simulink model "TEST1"  (R2023b)
settings: Solver=VariableStepAuto  StartTime=0.0  StopTime=10.0  RelTol=1e-3
libraries: spsExcitationSystemLib x2, spsMultiBandPowerSystemStabilizerLib x2, spsSynchronousMachinepuStandardLib x2, spsSteamTurbineandGovernorLib x2, spsThreePhaseTransformerTwoWindingsLib x2, spsThreePhasePISectionLineLib x2, spsThreePhaseParallelRLCLoadLib x1, sps_lib x1
settings Model: Creator=rohith  LastModifiedBy=rohith

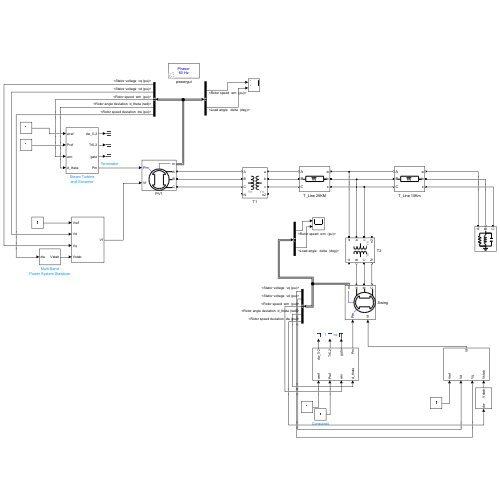
[thumbnail: Simulink's stored preview of the top-level diagram]
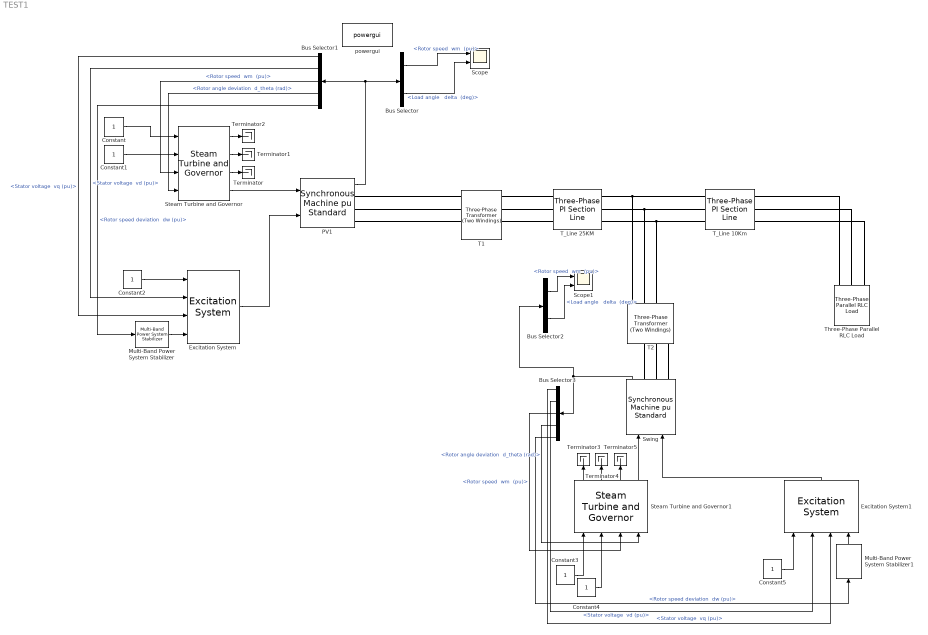
== system TEST1 ==
  Bus Selector : BusSelector  OutputSignals="Mechanical.Rotor speed  wm  (pu),Load angle   delta  (deg)"
  Bus Selector1 : BusSelector  OutputSignals="dq0 components.Stator voltage  vq (pu),dq0 components.Stator voltage  vd (pu),Mechanical.Rotor speed  wm  (pu),Mechanical.Rotor angle deviation  d_theta (rad),Mechanical.Rotor speed deviation  dw (pu)"
  Bus Selector2 : BusSelector  OutputSignals="Mechanical.Rotor speed  wm  (pu),Load angle   delta  (deg)"
  Bus Selector3 : BusSelector  OutputSignals="dq0 components.Stator voltage  vq (pu),dq0 components.Stator voltage  vd (pu),Mechanical.Rotor speed  wm  (pu),Mechanical.Rotor angle deviation  d_theta (rad),Mechanical.Rotor speed deviation  dw (pu)"
  Constant{,1..5} (6 alike) : Constant
  Excitation System : spsExcitationSystemLib/Excitation System  tr=20e-3  reg=[ 300, 0.001 ]  exc=[ 1, 0 ]  tgr=[ 0, 0 ]  damp=[ 0.001, 0.1 ]  sat=[ 0, 0 ]  lim=[ -11.5, 11.5, 0 ]  v0="[1.0  1.28]"
      settings: LibrarySourceBlock=sps_lib/Electrical Machines/Synchronous Machine Control/Excitation System
  Excitation System1 : spsExcitationSystemLib/Excitation System  tr=20e-3  reg=[ 300, 0.001 ]  exc=[ 1, 0 ]  tgr=[ 0, 0 ]  damp=[ 0.001, 0.1 ]  sat=[ 0, 0 ]  lim=[ -11.5, 11.5, 0 ]  v0="[1.0  1.28]"
      settings: LibrarySourceBlock=sps_lib/Electrical Machines/Synchronous Machine Control/Excitation System
  Multi-Band Power System Stabilizer : spsMultiBandPowerSystemStabilizerLib/Multi-Band Power System Stabilizer  OperationMode=Simplified settings  Kg=1.0  GL=[0.2 20]  GI=[0.9 25]  GH=[12.0 145]  GLd=[66 66 9.4]  TcLF=[1.667 2 0 0 0 0 2 2.4 0 0 0 0 1 1]  GId=[66 66 47.6]  TcIF=[1 1 0.25 0.3 0 0 1 1 0.3 0.36 0 0 0 0]  GHd=[66 66 233]  TcHF="[0.01 0.012 0 0 0 0  0.012 0.0144 0 0 0 0 1 1]"  LIM=[.075 .15 .15 .15]  Plot_On=off  MagdB_On=off  FreqRange=logspace(-2,2,500)
      settings: LibrarySourceBlock=|
      | sps_lib/Electrical Machines/Synchronous Machine Control/Multi-Band
      | Power System Stabilizer
  Multi-Band Power System Stabilizer1 : spsMultiBandPowerSystemStabilizerLib/Multi-Band Power System Stabilizer  OperationMode=Simplified settings  Kg=1.0  GL=[0.2 20]  GI=[0.9 25]  GH=[12.0 145]  GLd=[66 66 9.4]  TcLF=[1.667 2 0 0 0 0 2 2.4 0 0 0 0 1 1]  GId=[66 66 47.6]  TcIF=[1 1 0.25 0.3 0 0 1 1 0.3 0.36 0 0 0 0]  GHd=[66 66 233]  TcHF="[0.01 0.012 0 0 0 0  0.012 0.0144 0 0 0 0 1 1]"  LIM=[.075 .15 .15 .15]  Plot_On=off  MagdB_On=off  FreqRange=logspace(-2,2,500)
      settings: LibrarySourceBlock=|
      | sps_lib/Electrical Machines/Synchronous Machine Control/Multi-Band
      | Power System Stabilizer
  PV1 : spsSynchronousMachinepuStandardLib/Synchronous Machine pu Standard  PresetModel=No  MechanicalLoad=Mechanical power Pm  ShowDetailedParameters=on  RotorType=Round  Units=per unit standard parameters  MeasurementBus=off  NominalParameters=[900e6 20e3 60]  Reactances1=[ 1.81, 0.3, 0.23, 1.76, 0.65, 0.25, 0.15 ]  Reactances2=[2.24 0.17 0.12 1.02 0.13 0.08]  dAxisTimeConstants=Short-circuit  qAxisTimeConstants=Short-circuit  TimeConstants1="[ 4.4849  0.0681  0.1  ]"  TimeConstants2=[ 8.0, 0.03, 1.0, 0.07 ]  TimeConstants3="[  4.49  0.0681  0.0513  ]"  TimeConstants4=[ 8.0, 0.03, 0.3371, 0.0295 ]  TimeConstants5=[ 1.01, 0.053, 0.1 ]  TimeConstants6=[ 1.3201, 0.023, 1.0, 0.07 ]  TimeConstants7=[0.012 0.003 0.003]  TimeConstants8=[ 1.3201, 0.0231, 0.3371, 0.0295 ]  StatorResistance=0.037875  Mechanical=[0.1028 0.02056 2]  PolePairs=20  InitialConditions="[ 0  0  0  0  0  0  0  0  1 ]"  SetSaturation=on  Saturation=[0.6404,0.7127,0.8441,0.9214,0.9956,1.082,1.19,1.316,1.457;0.7,0.7698,0.8872,0.9466,0.9969,1.046,1.1,1.151,1.201]  LoadFlowParameters=[1,0,0,0,0]  TsPowergui=0  TsBlock=-1  IterativeModel=Trapezoidal non iterative  IterativeDiscreteModel=Trapezoidal non iterative  BusType=PV  Pref=700e3  Qref=0  Qmin=-inf  Qmax=inf  PLF=0  QLF=0
  Scope : Scope  NumInputPorts=2
  Scope1 : Scope  NumInputPorts=2
  Steam Turbine and Governor : spsSteamTurbineandGovernorLib/Steam Turbine and Governor  gentype=Tandem-compound (multi-mass)  reg1="[ 1  0.05    0 ]"  reg2="[ 0.001  0.15 ]"  reg3="[ -0.1  0.1  0  4.496]"  N=3600  turb1="[ 0  10   3.3   0.5   ]"  turb2="[ 0.5   0.5   0  0 ]"  HA="[  1.5498   0.24894  0  0 ]"  KA="[  83.47  42.702  0  0 ]"  DA="[  0.3104  0.05  0  0 ]*8"  ini1=250.35/555  ini2=[2.7247e-008,-120.13]
      settings: LibrarySourceBlock=|
      | sps_lib/Electrical Machines/Synchronous Machine Control/Steam Turbine
      | and Governor
  Steam Turbine and Governor1 : spsSteamTurbineandGovernorLib/Steam Turbine and Governor  gentype=Tandem-compound (multi-mass)  reg1="[ 1  0.05    0 ]"  reg2="[ 0.001  0.15 ]"  reg3="[ -0.1  0.1  0  4.496]"  N=3600  turb1="[ 0  10   3.3   0.5   ]"  turb2="[ 0.5   0.5   0  0 ]"  HA="[  1.5498   0.24894  0  0 ]"  KA="[  83.47  42.702  0  0 ]"  DA="[  0.3104  0.05  0  0 ]*8"  ini1=250.35/555  ini2=[2.7247e-008,-120.13]
      settings: LibrarySourceBlock=|
      | sps_lib/Electrical Machines/Synchronous Machine Control/Steam Turbine
      | and Governor
  Swing : spsSynchronousMachinepuStandardLib/Synchronous Machine pu Standard  PresetModel=No  MechanicalLoad=Mechanical power Pm  ShowDetailedParameters=on  RotorType=Round  Units=per unit standard parameters  MeasurementBus=off  NominalParameters=[900e6 20e3 60]  Reactances1=[ 1.81, 0.3, 0.23, 1.76, 0.65, 0.25, 0.15 ]  Reactances2=[2.24 0.17 0.12 1.02 0.13 0.08]  dAxisTimeConstants=Short-circuit  qAxisTimeConstants=Short-circuit  TimeConstants1="[ 4.4849  0.0681  0.1  ]"  TimeConstants2=[ 8.0, 0.03, 1.0, 0.07 ]  TimeConstants3="[  4.49  0.0681  0.0513  ]"  TimeConstants4=[ 8.0, 0.03, 0.3371, 0.0295 ]  TimeConstants5=[ 1.01, 0.053, 0.1 ]  TimeConstants6=[ 1.3201, 0.023, 1.0, 0.07 ]  TimeConstants7=[0.012 0.003 0.003]  TimeConstants8=[ 1.3201, 0.0231, 0.3371, 0.0295 ]  StatorResistance=0.037875  Mechanical=[0.1028 0.02056 2]  PolePairs=20  InitialConditions="[ 0  0  0  0  0  0  0  0  1 ]"  SetSaturation=on  Saturation=[0.6404,0.7127,0.8441,0.9214,0.9956,1.082,1.19,1.316,1.457;0.7,0.7698,0.8872,0.9466,0.9969,1.046,1.1,1.151,1.201]  LoadFlowParameters=[1,0,0,0,0]  TsPowergui=0  TsBlock=-1  IterativeModel=Trapezoidal non iterative  IterativeDiscreteModel=Trapezoidal non iterative  BusType=PV  Pref=700e6  Qref=0  Qmin=-inf  Qmax=inf  PLF=0  QLF=0
  T1 : spsThreePhaseTransformerTwoWindingsLib/Three-Phase Transformer (Two Windings)  Winding1Connection=Yn  Winding2Connection=Yn  CoreType=Three single-phase transformers  SetSaturation=off  Hysteresis=off  DataFile='hysteresis'  SetInitialFlux=off  Measurements=None  UNITS=pu  NominalPower=[ 900e6 , 60 ]  Winding1=[ 20e3 , 1e-6 , 0 ]  Winding2=[230e3 , 1e-6 , 0.15 ]  Rm=500  Lm=500  L0=0.5  Saturation=[ 0,0 ; 0.0024,1.2 ; 1.0,1.52 ]  InitialFluxes=[ 0.8 , -0.8 , 0.7 ]  BreakLoop=off  DiscreteSolver=Trapezoidal iterative  DataType=off  TransfoNumber=1
  T2 : spsThreePhaseTransformerTwoWindingsLib/Three-Phase Transformer (Two Windings)  Winding1Connection=Yn  Winding2Connection=Yn  CoreType=Three single-phase transformers  SetSaturation=off  Hysteresis=off  DataFile='hysteresis'  SetInitialFlux=off  Measurements=None  UNITS=pu  NominalPower=[ 900e6 , 60 ]  Winding1=[ 20e3 , 1e-6 , 0 ]  Winding2=[230e3 , 1e-6 , 0.15 ]  Rm=500  Lm=500  L0=0.5  Saturation=[ 0,0 ; 0.0024,1.2 ; 1.0,1.52 ]  InitialFluxes=[ 0.8 , -0.8 , 0.7 ]  BreakLoop=off  DiscreteSolver=Trapezoidal iterative  DataType=off  TransfoNumber=1
  T_Line 10Km : spsThreePhasePISectionLineLib/Three-Phase PI Section Line  LConnTagsString=a|b|c  RConnTagsString=A|B|C  Length=10  Frequency=60  Resistances=[ 0.0001*529 1.6]  Inductances="[ 0.001*529/377  0.0061]"  Capacitances=[0.00175/529/377 5.2489e-9]
  T_Line 25KM : spsThreePhasePISectionLineLib/Three-Phase PI Section Line  LConnTagsString=a|b|c  RConnTagsString=A|B|C  Length=25  Frequency=60  Resistances=[ 0.0001*529 1.6]  Inductances="[ 0.001*529/377  0.0061]"  Capacitances=[0.00175/529/377 5.2489e-9]
  Terminator{,1..5} (6 alike) : Terminator
  Three-Phase Parallel RLC Load : spsThreePhaseParallelRLCLoadLib/Three-Phase Parallel RLC Load  LConnTagsString=A|B|C  Configuration=Y (grounded)  NominalVoltage=230e3  Vabc=[1e3 1e3 1e3]  Vabcp=[1e3 1e3 1e3]  NominalFrequency=60  UnbalancedPower=off  ActivePower=967e6  InductivePower=100e6  CapacitivePower=187e6  Pabc=[10e3 9e3 11e3]  QLabc=[100 90 110]  QCabc=[100 90 110]  Pabcp=[10e3 9e3 11e3]  QLabcp=[100 90 110]  QCabcp=[100 90 110]  Measurements=None  LoadType=constant Z
  powergui : sps_lib/powergui  Priority=1  SimulationMode=Phasor  SampleTime=50e-6  frequency=60  Iterations=50  frequencyindice=60  Pbase=100e6  ErrMax=1e-4  UnitsV=kV  UnitsW=MW  buscounter=0  FunctionMessages=off  echomessages=off  EnableUseOfTLC=off  CurrentSourceSwitches=off  DisableSnubberDevices=off  DisableRonSwitches=off  DisableVfSwitches=off  DisplayEquations=off  AutomaticDiscreteSolvers=off  SolverType=Tustin/Backward Euler (TBE)  Interpol=off  ExternalGateDelay=off  methode=off  Ts=100  x0status=blocks  SPID=on  SwTol=0  HookPort=off  NonlinearTolerance=1e-4  nMaxIteration=100  ContinueOnMaxIteration=off  RestoreLinks=warning  ResistiveCurrentMeasurement=off  Frange=[0:2:500]  Ylog=off  Xlog=on  ShowGrid=off  save=off  variable=ZData  structure=0  ZoomFFT=off  StartTime=0.0  cycles=1  DisplayStyle=1  fundamental=60  FreqAxis=off  MaxFrequency=1000  frequencyindicesteady=1  RmsSteady=1  display=off
  wires:
  PV1/1 -> Bus Selector1/1, Bus Selector/1
  Steam Turbine and Governor/4 -> PV1/1
  Excitation System/1 -> PV1/2
  Steam Turbine and Governor1/4 -> Swing/1
  Excitation System1/1 -> Swing/2
  Constant/1 -> Steam Turbine and Governor/1
  Constant1/1 -> Steam Turbine and Governor/2
  Steam Turbine and Governor/3 -> Terminator/1
  Steam Turbine and Governor/2 -> Terminator1/1
  Steam Turbine and Governor/1 -> Terminator2/1
  Bus Selector1/1 -> Excitation System/3  "<Stator voltage  vq (pu)>"
  Bus Selector1/2 -> Excitation System/2  "<Stator voltage  vd (pu)>"
  Bus Selector1/3 -> Steam Turbine and Governor/3  "<Rotor speed  wm  (pu)>"
  Bus Selector1/4 -> Steam Turbine and Governor/4  "<Rotor angle deviation  d_theta (rad)>"
  Constant2/1 -> Excitation System/1
  Multi-Band Power System Stabilizer/1 -> Excitation System/4
  Bus Selector/1 -> Scope/1  "<Rotor speed  wm  (pu)>"
  Bus Selector/2 -> Scope/2  "<Load angle   delta  (deg)>"
  Swing/1 -> Bus Selector3/1, Bus Selector2/1
  Bus Selector3/1 -> Excitation System1/3  "<Stator voltage  vq (pu)>"
  Bus Selector3/2 -> Excitation System1/2  "<Stator voltage  vd (pu)>"
  Bus Selector3/3 -> Steam Turbine and Governor1/3  "<Rotor speed  wm  (pu)>"
  Bus Selector3/4 -> Steam Turbine and Governor1/4  "<Rotor angle deviation  d_theta (rad)>"
  Steam Turbine and Governor1/1 -> Terminator3/1
  Steam Turbine and Governor1/2 -> Terminator4/1
  Steam Turbine and Governor1/3 -> Terminator5/1
  Constant3/1 -> Steam Turbine and Governor1/1
  Constant4/1 -> Steam Turbine and Governor1/2
  Constant5/1 -> Excitation System1/1
  Bus Selector2/1 -> Scope1/1  "<Rotor speed  wm  (pu)>"
  Bus Selector2/2 -> Scope1/2  "<Load angle   delta  (deg)>"
  Bus Selector1/5 -> Multi-Band Power System Stabilizer/1  "<Rotor speed deviation  dw (pu)>"
  Multi-Band Power System Stabilizer1/1 -> Excitation System1/4
  Bus Selector3/5 -> Multi-Band Power System Stabilizer1/1  "<Rotor speed deviation  dw (pu)>"
  connections:
  PV1/RConn3 -- T1/LConn3
  PV1/RConn2 -- T1/LConn2
  PV1/RConn1 -- T1/LConn1
  T2/LConn3 -- Swing/RConn2
  Swing/RConn1 -- T2/LConn2
  Swing/RConn3 -- T2/LConn4
  T_Line 25KM/LConn2 -- T1/RConn2
  T1/RConn3 -- T_Line 25KM/LConn3
  T1/RConn1 -- T_Line 25KM/LConn1
  T_Line 10Km/LConn1 -- T_Line 25KM/RConn1 -- T2/RConn1
  T_Line 25KM/RConn2 -- T2/RConn2 -- T_Line 10Km/LConn2
  T_Line 25KM/RConn3 -- T2/RConn3 -- T_Line 10Km/LConn3
  T_Line 10Km/RConn1 -- Three-Phase Parallel RLC Load/LConn1
  Three-Phase Parallel RLC Load/LConn2 -- T_Line 10Km/RConn2
  T_Line 10Km/RConn3 -- Three-Phase Parallel RLC Load/LConn3
